simulink model "test"  (R2018b)
settings: Solver=FixedStepAuto  StartTime=0.0  StopTime=250  FixedStep=0.001  RelTol=1e-3
settings Model: Creator=User  LastModifiedBy=User

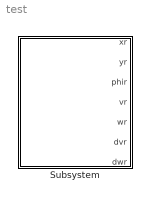
== system test ==
  Subsystem : Subsystem

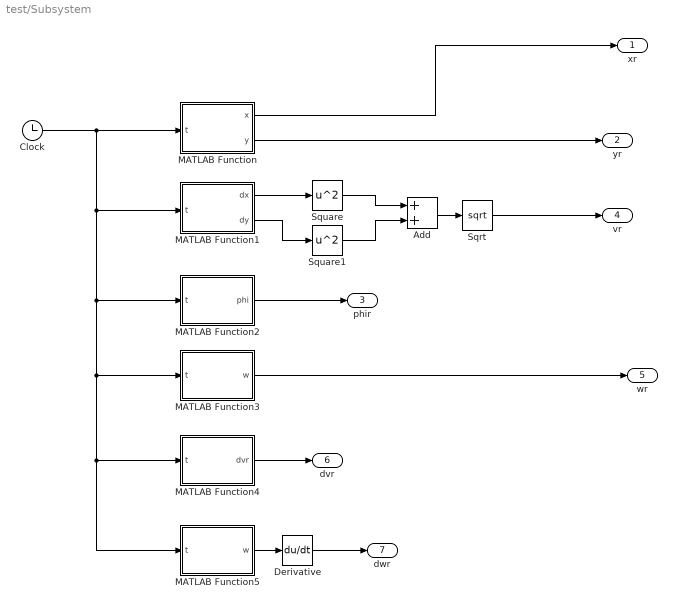
== system test/Subsystem ==
  Add : Sum
  Clock : Clock
  Derivative : Derivative
  MATLAB Function : MATLAB Function  TreatAsAtomicUnit=on
  MATLAB Function1 : MATLAB Function  TreatAsAtomicUnit=on
  MATLAB Function2 : MATLAB Function  TreatAsAtomicUnit=on
  MATLAB Function3 : MATLAB Function  TreatAsAtomicUnit=on
  MATLAB Function4 : MATLAB Function  TreatAsAtomicUnit=on
  MATLAB Function5 : MATLAB Function  TreatAsAtomicUnit=on
  Sqrt : Sqrt  SaturateOnIntegerOverflow=on
  Square : Math  Operator=square  SaturateOnIntegerOverflow=on
  Square1 : Math  Operator=square  SaturateOnIntegerOverflow=on
  xr : Outport
  yr : Outport  Port=2
  phir : Outport  Port=3
  vr : Outport  Port=4
  wr : Outport  Port=5
  dvr : Outport  Port=6
  dwr : Outport  Port=7
  wires:
  Add/1 -> Sqrt/1
  MATLAB Function3/1(w) -> wr/1
  MATLAB Function1/1(dx) -> Square/1
  MATLAB Function/2(y) -> yr/1
  MATLAB Function/1(x) -> xr/1
  MATLAB Function2/1(phi) -> phir/1
  Clock/1 -> MATLAB Function4/1(t), MATLAB Function5/1(t), MATLAB Function3/1(t), MATLAB Function2/1(t), MATLAB Function1/1(t), MATLAB Function/1(t)
  Square1/1 -> Add/2
  Square/1 -> Add/1
  MATLAB Function1/2(dy) -> Square1/1
  Sqrt/1 -> vr/1
  MATLAB Function4/1(dvr) -> dvr/1
  MATLAB Function5/1(w) -> Derivative/1
  Derivative/1 -> dwr/1

== matlab function test/Subsystem/MATLAB Function1 ==
  data: dx output; t input; dy output
function [dx,dy] = fcn(t)
dx=0;
dy=0;
if t<50
    dx=-2*pi/25*sin(pi/25*t);
    dy=2*pi/25*cos(pi/25*t);
elseif t<75
    dx=2*2*pi/25*sin(2*pi/25*(t-50));
    dy=2*2*pi/25*cos(2*pi/25*(t-50));
elseif t<100
    dx=-2*pi/25*sin(pi/25*(t-75));
    dy=2*pi/25*cos(pi/25*(t-75));
elseif t<130
    dx=-0.2;
    dy=0;
elseif t<150
    dx=-0.5;
    dy=pi/10*cos(pi/10*(t-130));
else 
    dx=10*pi/100*sin(pi/100*(t-150));
    dy=10*pi/100*cos(pi/100*(t-150));
end

== matlab function test/Subsystem/MATLAB Function ==
  data: x output; t input; y output
function [x,y] = fcn(t)
x=0;
y=0;
if t<50
    x=2*cos(pi/25*t);
    y=2*sin(pi/25*t);
elseif t<75
    x=4-2*cos(2*pi/25*(t-50));
    y=2*sin(2*pi/25*(t-50));
elseif t<100
    x=2*cos(pi/25*(t-75));
    y=2*sin(pi/25*(t-75));
elseif t<130
    x=-2-0.2*(t-100);
    y=0;
elseif t<150
    x=-8-0.5*(t-130);
    y=sin(pi/10*(t-130));
else 
    x=-8-10*cos(pi/100*(t-150));
    y=10*sin(pi/100*(t-150));
end

== matlab function test/Subsystem/MATLAB Function2 ==
  data: t input; phi output
function phi = fcn(t)
if t<50
    phi=pi/2+pi/25*t;
elseif t<75
    phi=5*pi/2-2*pi/25*(t-50);
elseif t<100
    phi=pi/2+pi/25*(t-75);
elseif t<130
    phi=pi;
elseif t<150
    phi=pi+atan(pi/10*cos(pi/10*(t-130))/-0.5);
else 
    phi=pi/2-pi/100*(t-150);
end
end

== matlab function test/Subsystem/MATLAB Function3 ==
  data: t input; w output
function w = fcn(t)
if t<50
    w=pi/25;
elseif t<75
    w=-2*pi/25;
elseif t<100
    w=pi/25;
elseif t<130
    w=0;
elseif t<150
    w=1/(1+(pi/10*cos(pi/10*(t-130))/-0.5)^2)*pi/10/0.5*sin(pi/10*(t-130))*pi/10;
else 
    w=-pi/100;
end
end

== matlab function test/Subsystem/MATLAB Function4 ==
  data: t input; dvr output
function dvr = fcn(t)
if t<50
    dvr=0;
elseif t<75
    dvr=0;
elseif t<100
    dvr=0;
elseif t<130
    dvr=0;
elseif t<150
    dvr=1/sqrt(0.25+(pi/10*cos(pi/10*(t-130)))^2)/2*2*(pi/10*cos(pi/10*(t-130)))*-pi/10*pi/10*sin(pi/10*(t-130));
else 
    dvr=0;
end
end

== matlab function test/Subsystem/MATLAB Function5 ==
  data: t input; w output
function w = fcn(t)
if t<50
    w=0;
elseif t<75
    w=0;
elseif t<100
    w=0;
elseif t<130
    w=0;
elseif t<150
    w=1/(1+(pi/10*cos(pi/10*(t-130))/-0.5)^2)*pi/10/0.5*sin(pi/10*(t-130))*pi/10;
else 
    w=0;
end
end
